simulink model "F_8g"  (R2017a)
settings: Solver=VariableStepAuto  StartTime=0.0  StopTime=100  RelTol=1e-3
undefined symbols (not defined in the file or in its folder): F_animation, P
libraries: simulink x1
settings Model: Creator=Mat Haskell  LastModifiedBy=Mat Haskell

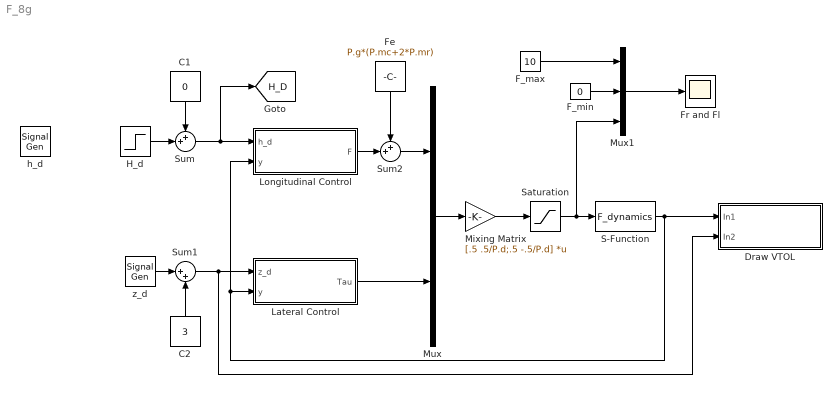
== system F_8g ==
  C1 : Constant  Value=0
  C2 : Constant  Value=3
  Draw VTOL : Subsystem
  F_max : Constant  Value=10
  F_min : Constant  Value=0
  Fe : Constant  Value=P.g*(P.mc+2*P.mr)
  Fr and Fl : Scope
  H_d : Step  Time=0  SampleTime=0
  Lateral Control : Subsystem
  Longitudinal Control : Subsystem
  Mixing Matrix : Gain  Gain=[.5 .5/P.d;.5 -.5/P.d]  Multiplication=Matrix(K*u)
  Mux : Mux  Inputs=2
  Mux1 : Mux  Inputs=3
  S-Function : S-Function  FunctionName=F_dynamics  Parameters=P  SFunctionDeploymentMode=off  EnableBusSupport=off
  Saturation : Saturate  UpperLimit=10  LowerLimit=0
  Sum : Sum  Inputs=++|
  Sum1 : Sum  Inputs=|++
  Sum2 : Sum  Inputs=++|
  h_d : SignalGenerator  WaveForm=square  Amplitude=0  Frequency=.08  Units=rad/sec
  z_d : SignalGenerator  WaveForm=square  Amplitude=2.5  Frequency=.08  Units=rad/sec
  tag scope: H_D=global
  wires:
  C1/1 -> Sum/1
  Sum/1 -> [H_D], Longitudinal Control/1(h_d)
  z_d/1 -> Sum1/1
  C2/1 -> Sum1/2
  Sum1/1 -> Draw VTOL/2(In2), Lateral Control/1(z_d)
  Lateral Control/1(Tau) -> Mux/2
  Mux/1 -> Mixing Matrix/1
  S-Function/1 -> Draw VTOL/1(In1), Longitudinal Control/2("y "), Lateral Control/2("y ")
  Longitudinal Control/1(F) -> Sum2/2
  Sum2/1 -> Mux/1
  Fe/1 -> Sum2/1
  H_d/1 -> Sum/2
  Mixing Matrix/1 -> Saturation/1
  Mux1/1 -> Fr and Fl/1
  F_min/1 -> Mux1/2
  F_max/1 -> Mux1/1
  Saturation/1 -> Mux1/3, S-Function/1

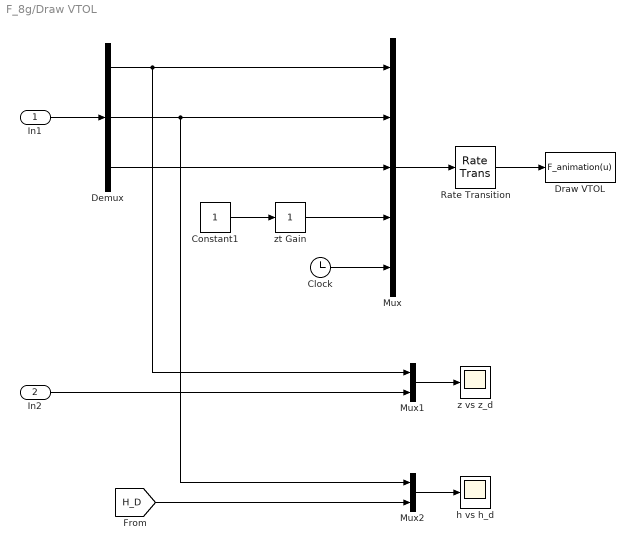
== system F_8g/Draw VTOL ==
  In1 : Inport
  In2 : Inport  Port=2
  Clock : Clock
  Constant1 : Constant
  Demux : Demux  Outputs=3
  Draw VTOL : MATLABFcn  InitFcn=|  MATLABFcn=F_animation(u)  OutputDimensions=0
      | clear;clc
      | F_param
  Mux : Mux  Inputs=5
  Mux1 : Mux  Inputs=2
  Mux2 : Mux  Inputs=2
  Rate Transition : RateTransition  OutPortSampleTime=P.t_plot
  h vs h_d : Scope
  z vs z_d : Scope
  zt Gain : simulink/Math Operations/Slider Gain  gain=1  low=0  high=5
  wires:
  In1/1 -> Demux/1
  Demux/1 -> Mux1/1, Mux/1
  Demux/2 -> Mux2/1, Mux/2
  Demux/3 -> Mux/3
  Rate Transition/1 -> Draw VTOL/1
  Mux/1 -> Rate Transition/1
  zt Gain/1 -> Mux/4
  Constant1/1 -> zt Gain/1
  Clock/1 -> Mux/5
  In2/1 -> Mux1/2
  Mux1/1 -> z vs z_d/1
  Mux2/1 -> h vs h_d/1
  [H_D] -> Mux2/2

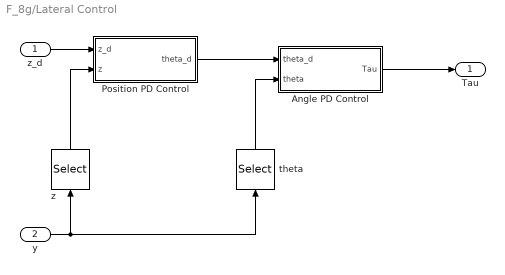
== system F_8g/Lateral Control ==
  z_d : Inport
  "y " : Inport  Port=2
  Angle PD Control : Subsystem
  Position PD Control : Subsystem
  theta : Selector  InputPortWidth=3  IndexOptions=Index vector (dialog)  Indices=[3]  OutputSizes=1
  z : Selector  InputPortWidth=3  IndexOptions=Index vector (dialog)  Indices=[1]  OutputSizes=1
  Tau : Outport
  wires:
  z_d/1 -> Position PD Control/1(z_d)
  "y "/1 -> theta/1, z/1
  z/1 -> Position PD Control/2(z)
  Position PD Control/1(theta_d) -> Angle PD Control/1(theta_d)
  theta/1 -> Angle PD Control/2(theta)
  Angle PD Control/1(Tau) -> Tau/1

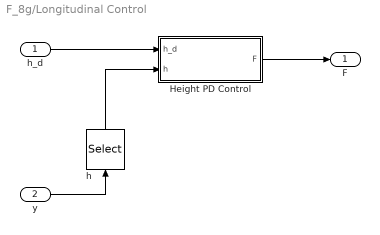
== system F_8g/Longitudinal Control ==
  h_d : Inport
  "y " : Inport  Port=2
  Height PD Control : Subsystem
  h : Selector  InputPortWidth=3  IndexOptions=Index vector (dialog)  Indices=[2]  OutputSizes=1
  F : Outport
  wires:
  h_d/1 -> Height PD Control/1(h_d)
  Height PD Control/1(F) -> F/1
  "y "/1 -> h/1
  h/1 -> Height PD Control/2(h)

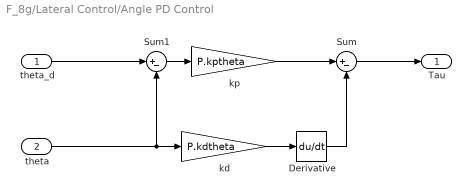
== system F_8g/Lateral Control/Angle PD Control ==
  theta_d : Inport
  theta : Inport  Port=2
  Derivative : Derivative
  Sum : Sum  Inputs=|+-
  Sum1 : Sum  Inputs=|+-
  kd : Gain  Gain=P.kdtheta
  kp : Gain  Gain=P.kptheta
  Tau : Outport
  wires:
  Derivative/1 -> Sum/2
  Sum1/1 -> kp/1
  theta_d/1 -> Sum1/1
  Sum/1 -> Tau/1
  kp/1 -> Sum/1
  kd/1 -> Derivative/1
  theta/1 -> Sum1/2, kd/1

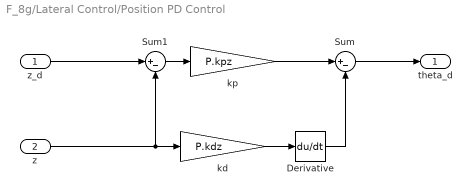
== system F_8g/Lateral Control/Position PD Control ==
  z_d : Inport
  z : Inport  Port=2
  Derivative : Derivative
  Sum : Sum  Inputs=|+-
  Sum1 : Sum  Inputs=|+-
  kd : Gain  Gain=P.kdz
  kp : Gain  Gain=P.kpz
  theta_d : Outport
  wires:
  Derivative/1 -> Sum/2
  Sum1/1 -> kp/1
  z_d/1 -> Sum1/1
  Sum/1 -> theta_d/1
  kp/1 -> Sum/1
  kd/1 -> Derivative/1
  z/1 -> Sum1/2, kd/1

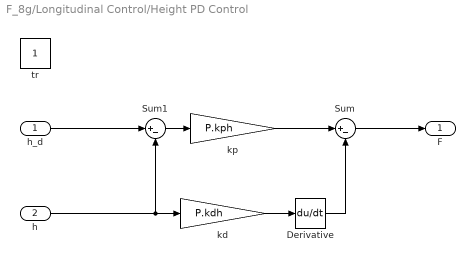
== system F_8g/Longitudinal Control/Height PD Control ==
  h_d : Inport
  h : Inport  Port=2
  Derivative : Derivative
  Sum : Sum  Inputs=|+-
  Sum1 : Sum  Inputs=|+-
  kd : Gain  Gain=P.kdh
  kp : Gain  Gain=P.kph
  tr : Constant
  F : Outport
  wires:
  Derivative/1 -> Sum/2
  Sum1/1 -> kp/1
  h_d/1 -> Sum1/1
  Sum/1 -> F/1
  kp/1 -> Sum/1
  kd/1 -> Derivative/1
  h/1 -> Sum1/2, kd/1
